simulink model "R3"  (R2018a)
settings: Solver=VariableStepAuto  StartTime=0.0  StopTime=100000  RelTol=1e-3
values from neighbouring files (symbols this model uses):
  k = log2(M)    [Code.m]
  U = zeros(1,M)    [Code.m]
  V = zeros(1,M)    [Code.m]
  W = zeros(1,M)    [Code.m]
libraries: commdigbbndam3 x2, commchan3 x1, commsink2 x1, commrandsrc3 x1
settings Model: Creator=Prof. S.R.Singh  LastModifiedBy=Prof. S.R.Singh

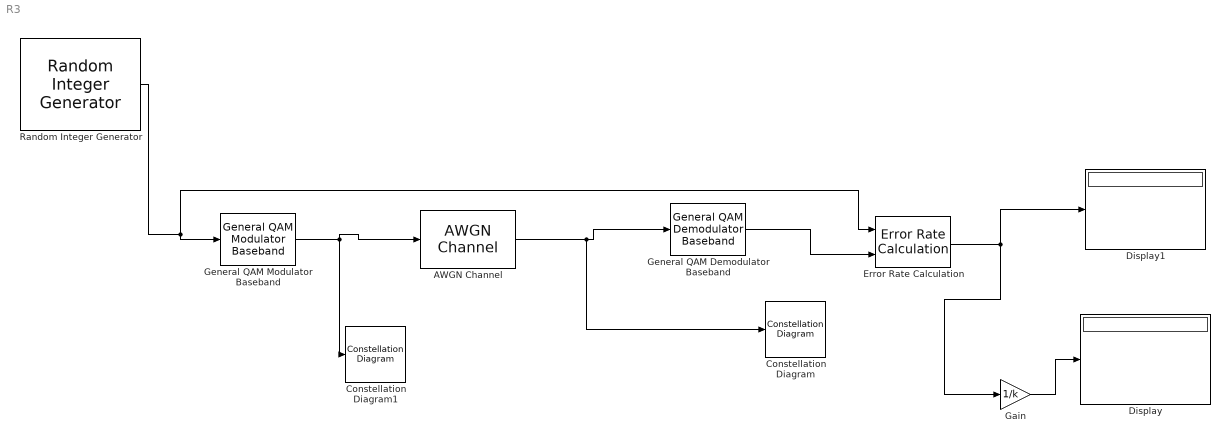
== system R3 ==
  AWGN Channel : commchan3/AWGN Channel  InputProcessing=Columns as channels (frame based)  seed=67  noiseMode="Signal to noise ratio  (Eb/No)"  EbNodB=5 + 10*log10(k)  EsNodB=10  SNRdB=10  bitsPerSym=1  Ps=1  Tsym=1  variance=1
  Constellation Diagram : ConstellationDiagram
  Constellation Diagram1 : ConstellationDiagram
  Display : Display
  Display1 : Display
      settings: Decimation=3
  Error Rate Calculation : commsink2/Error Rate Calculation  N=0  st_delay=0  cp_mode=Entire frame  subframe=[]  PMode=Port  WsName=ErrorVec  RsMode2=off  stop=off  numErr=100  maxBits=1e6
  Gain : Gain  Gain=1/k
  General QAM Demodulator Baseband : commdigbbndam3/General QAM Demodulator Baseband  SigCon=V.*[exp(2*pi*1i*(W./4+U) )]  OutType=Integer  DecType=Hard decision  VarSource=Dialog  Variance=1  outDtypeBit=Inherit via internal rule  outDtype=Inherit via internal rule  roundingMode=Floor  overflowMode=Wrap  OvFlMode=off  OvFlModeLastStrValue=off  sigConstWordLen=16  sigConstDataTypeStr=Inherit: Same word length as input  sigConstLastDataTypeStr=Inherit: Same word length as input  accum1WordLen=32  accum1FracLen=30  prodInWordLen=32  prodInFracLen=30  prodInDataTypeStr=Inherit: Same as accumulator 1  prodInLastDataTypeStr=Inherit: Same as accumulator 1  prodOutWordLen=32  prodOutFracLen=30  accum2WordLen=32  accum2FracLen=30  accum3WordLen=32  accum3FracLen=30  nsiWordLen=32  nsiFracLen=30  nsiDataTypeStr=Inherit: Same as accumulator 3  nsiLastDataTypeStr=Inherit: Same as accumulator 3  invn0WordLen=16  invn0FracLen=8  invn0DataTypeStr=Inherit: Same word length as input  invn0LastDataTypeStr=Inherit: Same word length as input  outputWordLen=32  outputFracLen=30
      settings: SourceProductName=Communications System Toolbox  SourceProductBaseCode=CM
  General QAM Modulator Baseband : commdigbbndam3/General QAM Modulator Baseband  SigCon=V.*[exp(2*pi*1i*(W./4+U) )]  outDtype=double  outWordLen=16  outUDDataType=sfix(16)  outFracLenMode=Best precision  outFracLen=15  outDataTypeStr=double  outLastDataTypeStr=double
      settings: SourceProductName=Communications System Toolbox  SourceProductBaseCode=CM
  Random Integer Generator : commrandsrc3/Random Integer Generator  SetSize=M  SeedSource=Parameter  Seed=37  SampleTime=1  SamplesPerFrame=1  OutputDataType=double  SimulateUsing=Interpreted execution
  wires:
  General QAM Modulator Baseband/1 -> AWGN Channel/1, Constellation Diagram1/1
  Error Rate Calculation/1 -> Display1/1, Gain/1
  AWGN Channel/1 -> General QAM Demodulator Baseband/1, Constellation Diagram/1
  Gain/1 -> Display/1
  General QAM Demodulator Baseband/1 -> Error Rate Calculation/2
  Random Integer Generator/1 -> General QAM Modulator Baseband/1, Error Rate Calculation/1
